simulink model "Inv_Pend_PID5"  (R2023b)
settings: Solver=VariableStepAuto  StartTime=0.0  StopTime=50  RelTol=1e-3
values from neighbouring files (symbols this model uses):
  b = 0.1    [Parameters.m]    (also in Parameters3.m; Parameters_Tf.m)
  g = 9.81    [Parameters.m]    (also in Parameters3.m = 9.8; Parameters_Tf.m = 9.8)
  J = 0.006    [Parameters.m]    (also in Parameters_Tf.m)
  L = 0.3    [Parameters.m]    (also in Parameters3.m = 0.5; Parameters_Tf.m)
  M = 0.5    [Parameters.m]    (also in Parameters3.m = 2; Parameters_Tf.m)
  m = 0.2    [Parameters.m]    (also in Parameters3.m; Parameters_Tf.m = 0.3)
libraries: slpidlib x2
settings Model: Creator=DELL  LastModifiedBy=DELL

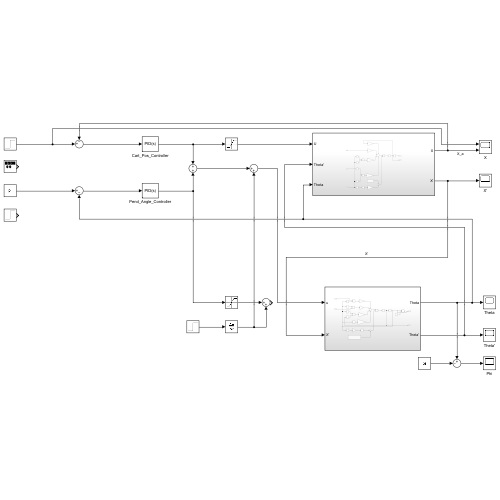
[thumbnail: Simulink's stored preview of the top-level diagram]
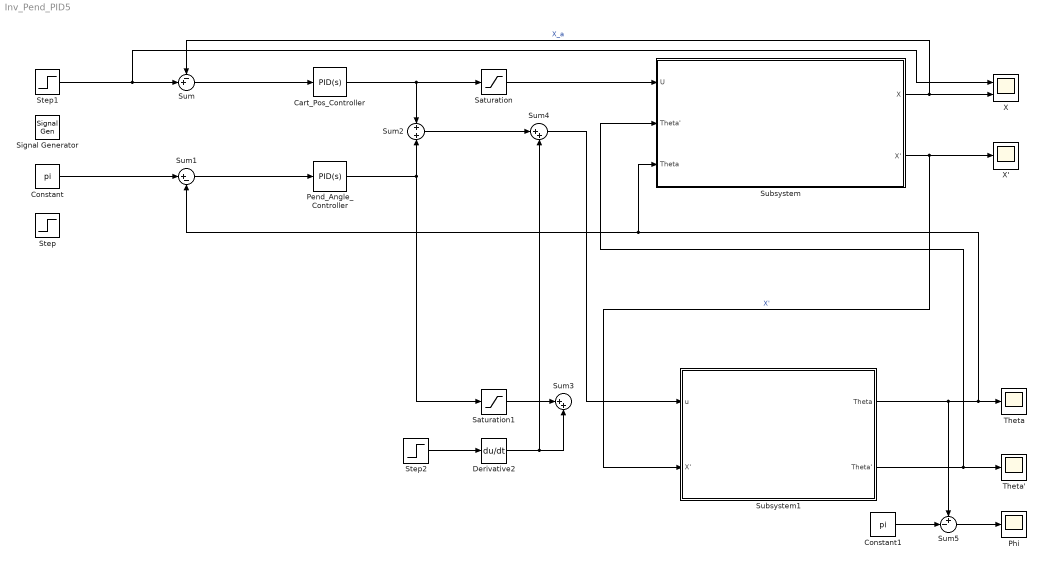
== system Inv_Pend_PID5 ==
  Cart_Pos_Controller : slpidlib/PID Controller  Controller=PID  Form=Parallel  TimeDomain=Continuous-time  UseExternalTs=off  SampleTime=-1  IntegratorMethod=Forward Euler  FilterMethod=Forward Euler  ControllerParametersSource=internal  P=-1.5  I=0  UseKiTs=off  D=-3.6  N=121.318437755644  UseFilter=on  TunerSelectOption=Transfer Function Based (PID Tuner App)  InitialConditionSource=internal  InitialConditionForIntegrator=0  InitialConditionForFilter=0  DifferentiatorICPrevScaledInput=0  ExternalReset=none  TrackingMode=off  Kt=1  LimitOutput=off  SatLimitsSource=internal  UpperSaturationLimit=inf  LowerSaturationLimit=-inf  LinearizeAsGain=on  AntiWindupMode=none  Kb=1  LimitIntegrator=off  UpperIntegratorSaturationLimit=inf  LowerIntegratorSaturationLimit=-inf  POutMin=[]  POutMax=[]  IOutMin=[]  IOutMax=[]  DOutMin=[]  DOutMax=[]  NOutMin=[]  NOutMax=[]  SumOutMin=[]  SumOutMax=[]  SaturationOutMin=[]  SaturationOutMax=[]  PParamMin=[]  PParamMax=[]  IParamMin=[]  IParamMax=[]  DParamMin=[]  DParamMax=[]  NParamMin=[]  NParamMax=[]  KbParamMin=[]  KbParamMax=[]  KtParamMin=[]  KtParamMax=[]  KbOutMin=[]  KbOutMax=[]  KtOutMin=[]  KtOutMax=[]  IntegratorOutMin=[]  IntegratorOutMax=[]  FilterOutMin=[]  FilterOutMax=[]  SumI1OutMin=[]  SumI1OutMax=[]  SumI2OutMin=[]  SumI2OutMax=[]  SumI3OutMin=[]  SumI3OutMax=[]  SumI4OutMin=[]  SumI4OutMax=[]  SumDOutMin=[]  SumDOutMax=[]  DifferentiatorOutMin=[]  DifferentiatorOutMax=[]  FilterDiffOutCoefMin=[]  FilterDiffOutCoefMax=[]  ReciprocalOutMin=[]  ReciprocalOutMax=[]  SumDenOutMin=[]  SumDenOutMax=[]  SumNumOutMin=[]  SumNumOutMax=[]  DivideOutMin=[]  DivideOutMax=[]  UdiffTsProdOutMin=[]  UdiffTsProdOutMax=[]  NTsProdOutMin=[]  NTsProdOutMax=[]  UintegralTsProdOutMin=[]  UintegralTsProdOutMax=[]  UngainTsProdOutMin=[]  UngainTsProdOutMax=[]  ClampingZeroOutDataTypeStr=Inherit: Inherit via back propagation  ClampingZeroOutMin=[]  ClampingZeroOutMax=[]  FilterDenConstantOutDataTypeStr=Inherit: Inherit via back propagation  FilterDenConstantOutMin=[]  FilterDenConstantOutMax=[]  PCopyOutDataTypeStr=Inherit: Inherit via back propagation  PCopyOutMin=[]  PCopyOutMax=[]  NCopyOutDataTypeStr=Inherit: Inherit via back propagation  NCopyOutMin=[]  NCopyOutMax=[]  IntegratorContinuousStateAttributes=''  IntegratorStateMustResolveToSignalObject=off  IntegratorRTWStateStorageClass=Auto  FilterContinuousStateAttributes=''  FilterStateMustResolveToSignalObject=off  FilterRTWStateStorageClass=Auto  ParallelPVariant=InternalParameters  IdealPVariant=Disabled  IVariant=InternalParameters  DVariant=InternalParameters  IntegratorVariant=Continuous  SatVariant=Disabled  AWVariant=Passthrough  PCopyVariant=Disabled  TRVariant=Disabled  FdbkBlocksVariant=Forward  IdealPFdbkVariant=Disabled  SatFdbkVariant=Disabled  DerivativeFilterVariant=ContFilter  NVariant=InternalParameters  NCopyVariant=Disabled  FilterICVariant=InternalICsFilter  IntegratorICVariant=InternalICs  ExternalResetVariant=Disabled  TRSumVariant=Passthrough  SumFdbkVariant=Disabled  SumVariant=Sum_PID  TsampFilterVariant=InternalTs  TsampNgainVariant=Passthrough  TsampIntegralVariant=Disabled_SignalSpec  ExternalSaturationOutDataTypeStr=Inherit: Same as second input
  Constant : Constant  Value=pi
  Constant1 : Constant  Value=pi
  Derivative2 : Derivative
  Pend_Angle_Controller : slpidlib/PID Controller  Controller=PID  Form=Parallel  TimeDomain=Continuous-time  UseExternalTs=off  SampleTime=-1  IntegratorMethod=Forward Euler  FilterMethod=Forward Euler  ControllerParametersSource=internal  P=-30  I=0  UseKiTs=off  D=-10  N=39.9551478640311  UseFilter=on  TunerSelectOption=Transfer Function Based (PID Tuner App)  InitialConditionSource=internal  InitialConditionForIntegrator=0  InitialConditionForFilter=0  DifferentiatorICPrevScaledInput=0  ExternalReset=none  TrackingMode=off  Kt=1  LimitOutput=off  SatLimitsSource=internal  UpperSaturationLimit=inf  LowerSaturationLimit=-inf  LinearizeAsGain=on  AntiWindupMode=none  Kb=1  LimitIntegrator=off  UpperIntegratorSaturationLimit=inf  LowerIntegratorSaturationLimit=-inf  POutMin=[]  POutMax=[]  IOutMin=[]  IOutMax=[]  DOutMin=[]  DOutMax=[]  NOutMin=[]  NOutMax=[]  SumOutMin=[]  SumOutMax=[]  SaturationOutMin=[]  SaturationOutMax=[]  PParamMin=[]  PParamMax=[]  IParamMin=[]  IParamMax=[]  DParamMin=[]  DParamMax=[]  NParamMin=[]  NParamMax=[]  KbParamMin=[]  KbParamMax=[]  KtParamMin=[]  KtParamMax=[]  KbOutMin=[]  KbOutMax=[]  KtOutMin=[]  KtOutMax=[]  IntegratorOutMin=[]  IntegratorOutMax=[]  FilterOutMin=[]  FilterOutMax=[]  SumI1OutMin=[]  SumI1OutMax=[]  SumI2OutMin=[]  SumI2OutMax=[]  SumI3OutMin=[]  SumI3OutMax=[]  SumI4OutMin=[]  SumI4OutMax=[]  SumDOutMin=[]  SumDOutMax=[]  DifferentiatorOutMin=[]  DifferentiatorOutMax=[]  FilterDiffOutCoefMin=[]  FilterDiffOutCoefMax=[]  ReciprocalOutMin=[]  ReciprocalOutMax=[]  SumDenOutMin=[]  SumDenOutMax=[]  SumNumOutMin=[]  SumNumOutMax=[]  DivideOutMin=[]  DivideOutMax=[]  UdiffTsProdOutMin=[]  UdiffTsProdOutMax=[]  NTsProdOutMin=[]  NTsProdOutMax=[]  UintegralTsProdOutMin=[]  UintegralTsProdOutMax=[]  UngainTsProdOutMin=[]  UngainTsProdOutMax=[]  ClampingZeroOutDataTypeStr=Inherit: Inherit via back propagation  ClampingZeroOutMin=[]  ClampingZeroOutMax=[]  FilterDenConstantOutDataTypeStr=Inherit: Inherit via back propagation  FilterDenConstantOutMin=[]  FilterDenConstantOutMax=[]  PCopyOutDataTypeStr=Inherit: Inherit via back propagation  PCopyOutMin=[]  PCopyOutMax=[]  NCopyOutDataTypeStr=Inherit: Inherit via back propagation  NCopyOutMin=[]  NCopyOutMax=[]  IntegratorContinuousStateAttributes=''  IntegratorStateMustResolveToSignalObject=off  IntegratorRTWStateStorageClass=Auto  FilterContinuousStateAttributes=''  FilterStateMustResolveToSignalObject=off  FilterRTWStateStorageClass=Auto  ParallelPVariant=InternalParameters  IdealPVariant=Disabled  IVariant=InternalParameters  DVariant=InternalParameters  IntegratorVariant=Continuous  SatVariant=Disabled  AWVariant=Passthrough  PCopyVariant=Disabled  TRVariant=Disabled  FdbkBlocksVariant=Forward  IdealPFdbkVariant=Disabled  SatFdbkVariant=Disabled  DerivativeFilterVariant=ContFilter  NVariant=InternalParameters  NCopyVariant=Disabled  FilterICVariant=InternalICsFilter  IntegratorICVariant=InternalICs  ExternalResetVariant=Disabled  TRSumVariant=Passthrough  SumFdbkVariant=Disabled  SumVariant=Sum_PID  TsampFilterVariant=InternalTs  TsampNgainVariant=Passthrough  TsampIntegralVariant=Disabled_SignalSpec  ExternalSaturationOutDataTypeStr=Inherit: Same as second input
  Phi : Scope
  Saturation : Saturate  UpperLimit=50  LowerLimit=-50
  Saturation1 : Saturate  UpperLimit=50  LowerLimit=-50
  Signal Generator : SignalGenerator  Amplitude=0.5
  Step : Step  SampleTime=0
  Step1 : Step  After=5  SampleTime=0
  Step2 : Step  After=50  SampleTime=0
  Subsystem : Subsystem
  Subsystem1 : Subsystem
  Sum : Sum  Inputs=-+|
  Sum1 : Sum  Inputs=|+-
  Sum2 : Sum  Inputs=+|+
  Sum3 : Sum  Inputs=|++
  Sum4 : Sum  Inputs=|++
  Sum5 : Sum  Inputs=+-|
  Theta : Scope
  Theta' : Scope
  X : Scope  NumInputPorts=2
  X' : Scope
  wires:
  Sum1/1 -> Pend_Angle_Controller/1
  Sum/1 -> Cart_Pos_Controller/1
  Cart_Pos_Controller/1 -> Saturation/1, Sum2/1
  Subsystem/1(X) -> X/2, Sum/1  "X_a"
  Subsystem/2(X') -> X'/1, Subsystem1/2(X')  "X'"
  Subsystem1/2(Theta') -> Theta'/1, Subsystem/2(Theta')
  Subsystem1/1(Theta) -> Sum1/2, Subsystem/3(Theta), Theta/1, Sum5/1
  Step2/1 -> Derivative2/1
  Derivative2/1 -> Sum3/2, Sum4/2
  Pend_Angle_Controller/1 -> Saturation1/1, Sum2/2
  Saturation1/1 -> Sum3/1
  Step1/1 -> X/1, Sum/2
  Sum5/1 -> Phi/1
  Constant1/1 -> Sum5/2
  Constant/1 -> Sum1/1
  Sum4/1 -> Subsystem1/1(u)
  Sum2/1 -> Sum4/1
  Saturation/1 -> Subsystem/1(U)

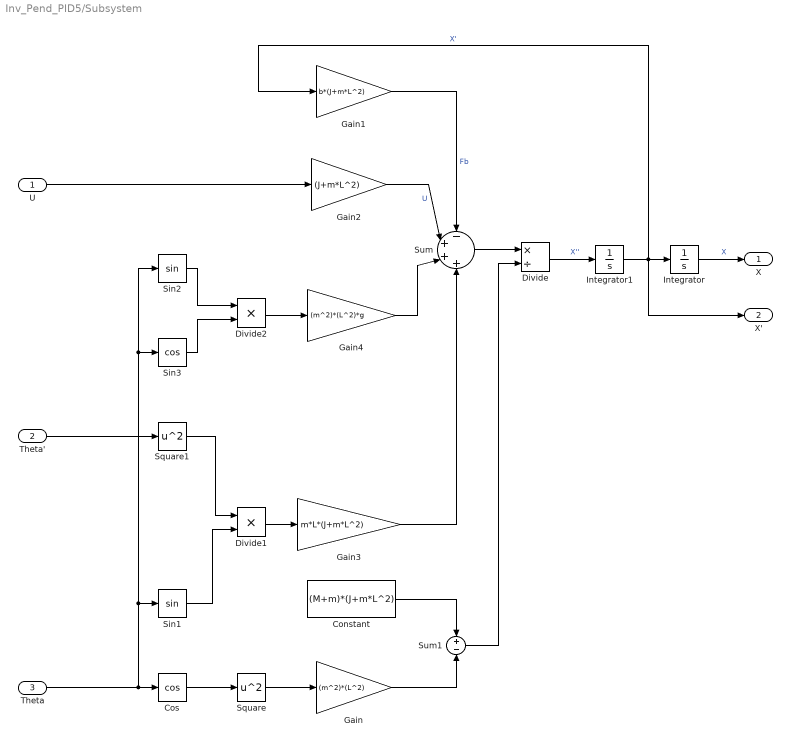
== system Inv_Pend_PID5/Subsystem ==
  U : Inport
  Theta' : Inport  Port=2
  Theta : Inport  Port=3
  Constant : Constant  Value=(M+m)*(J+m*L^2)
  Cos : Trigonometry  Operator=cos
  Divide : Product  Inputs=*/
  Divide1 : Product  Inputs=**
  Divide2 : Product  Inputs=**
  Gain : Gain  Gain=(m^2)*(L^2)
  Gain1 : Gain  Gain=b*(J+m*L^2)
  Gain2 : Gain  Gain=(J+m*L^2)
  Gain3 : Gain  Gain=m*L*(J+m*L^2)
  Gain4 : Gain  Gain=(m^2)*(L^2)*g
  Integrator : Integrator
  Integrator1 : Integrator
  Sin1 : Trigonometry
  Sin2 : Trigonometry
  Sin3 : Trigonometry  Operator=cos
  Square : Math  Operator=square
  Square1 : Math  Operator=square
  Sum : Sum  Inputs=-+++
  Sum1 : Sum  Inputs=+|-
  X : Outport
  X' : Outport  Port=2
  wires:
  Square/1 -> Gain/1
  Square1/1 -> Divide1/1
  Theta/1 -> Sin2/1, Sin3/1, Sin1/1, Cos/1
  Integrator1/1 -> X'/1, Gain1/1, Integrator/1  "X'"
  Constant/1 -> Sum1/1
  Divide/1 -> Integrator1/1  "X''"
  Sin1/1 -> Divide1/2
  Integrator/1 -> X/1  "X"
  Gain1/1 -> Sum/1  "Fb"
  Cos/1 -> Square/1
  Sum/1 -> Divide/1
  Divide2/1 -> Gain4/1
  Gain/1 -> Sum1/2
  Sin3/1 -> Divide2/2
  U/1 -> Gain2/1
  Sum1/1 -> Divide/2
  Sin2/1 -> Divide2/1
  Theta'/1 -> Square1/1
  Gain3/1 -> Sum/4
  Divide1/1 -> Gain3/1
  Gain4/1 -> Sum/3
  Gain2/1 -> Sum/2  "U"

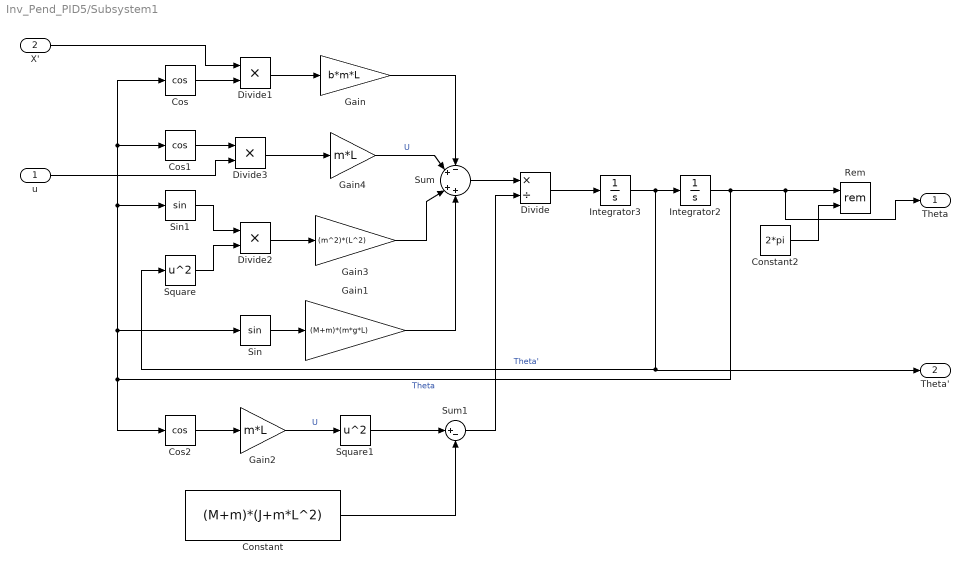
== system Inv_Pend_PID5/Subsystem1 ==
  u : Inport
  X' : Inport  Port=2
  Constant : Constant  Value=(M+m)*(J+m*L^2)
  Constant2 : Constant  Value=2*pi
  Cos : Trigonometry  Operator=cos
  Cos1 : Trigonometry  Operator=cos
  Cos2 : Trigonometry  Operator=cos
  Divide : Product  Inputs=*/
  Divide1 : Product  Inputs=**
  Divide2 : Product  Inputs=**
  Divide3 : Product  Inputs=**
  Gain : Gain  Gain=b*m*L
  Gain1 : Gain  Gain=(M+m)*(m*g*L)
  Gain2 : Gain  Gain=m*L
  Gain3 : Gain  Gain=(m^2)*(L^2)
  Gain4 : Gain  Gain=m*L
  Integrator2 : Integrator
  Integrator3 : Integrator
  Rem : Math  Operator=rem
  Sin : Trigonometry
  Sin1 : Trigonometry
  Square : Math  Operator=square
  Square1 : Math  Operator=square
  Sum : Sum  Inputs=-+|++
  Sum1 : Sum  Inputs=|+-
  Theta : Outport
  Theta' : Outport  Port=2
  wires:
  Gain4/1 -> Sum/2  "U"
  Square/1 -> Divide2/2
  Divide1/1 -> Gain/1
  Cos1/1 -> Divide3/1
  Sin/1 -> Gain1/1
  Divide2/1 -> Gain3/1
  Sin1/1 -> Divide2/1
  Divide3/1 -> Gain4/1
  Sum/1 -> Divide/1
  Divide/1 -> Integrator3/1
  Cos/1 -> Divide1/2
  Gain1/1 -> Sum/4
  Integrator2/1 -> Theta/1, Rem/1, Cos2/1, Sin/1, Cos/1, Cos1/1, Sin1/1  "Theta"
  u/1 -> Divide3/2
  X'/1 -> Divide1/1
  Integrator3/1 -> Square/1, Theta'/1, Integrator2/1  "Theta'"
  Gain2/1 -> Square1/1  "U"
  Cos2/1 -> Gain2/1
  Square1/1 -> Sum1/1
  Sum1/1 -> Divide/2
  Constant/1 -> Sum1/2
  Constant2/1 -> Rem/2
  Gain/1 -> Sum/1
  Gain3/1 -> Sum/3
